simulink model "solarMomentSimplified"  (R2023b)
settings: Solver=VariableStepAuto  StartTime=0.0  StopTime=Tfinal  RelTol=1e-3
model workspace (MAT data in the model file):
  I_sim = [38538.5406483  0  0; 0  45879.2150575  0; 0  0  36244.5798954]
  areas = [26.28; 12; 3; 7.5; 17.1; 53.96; 53.96; 4.5; 26.28; 20.1]
  centroids = [4.30109589041  0  1.69726027397; 8.04  1.25  2.4; 7.44  1.25  4.8; 0  1.25  1.5; 3.42  1.25  3; 4.02  9.6  2.3; 4.02  9.6  2.3; 6.84  1.25  3.9; 4.30109589041  0  1.69726027397; 4.02  1.25  0]
  normalVectors = [0  -1  0; 1  0  0; 0  0  1; -1  0  0; 0  0  1; 0  0  1; 0  0  -1; -1  0  0; 0  1  0; 0  0  -1]
  rcm = [4.05894270882 1.95833333333 1.80412649485]
values from neighbouring files (symbols this model uses):
  A_ptob = [0.00452111179393  0.994865050863  -0.101109297888; -0.99864921572  -0.000741813086313  -0.051953764597; -0.0517619888586  0.101207609816  0.993517848971]    [magConstants.mat]
libraries: vrlib x1
settings Model: Creator=kristopherriordan  LastModifiedBy=annahylbert
settings DebuggingCC: UnderSpecifiedDimensionMsg=warning

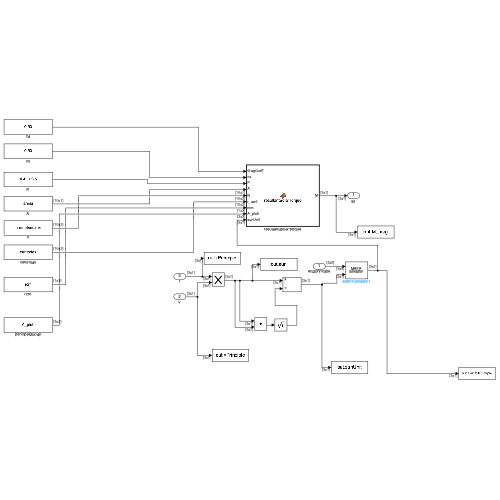
[thumbnail: Simulink's stored preview of the top-level diagram]
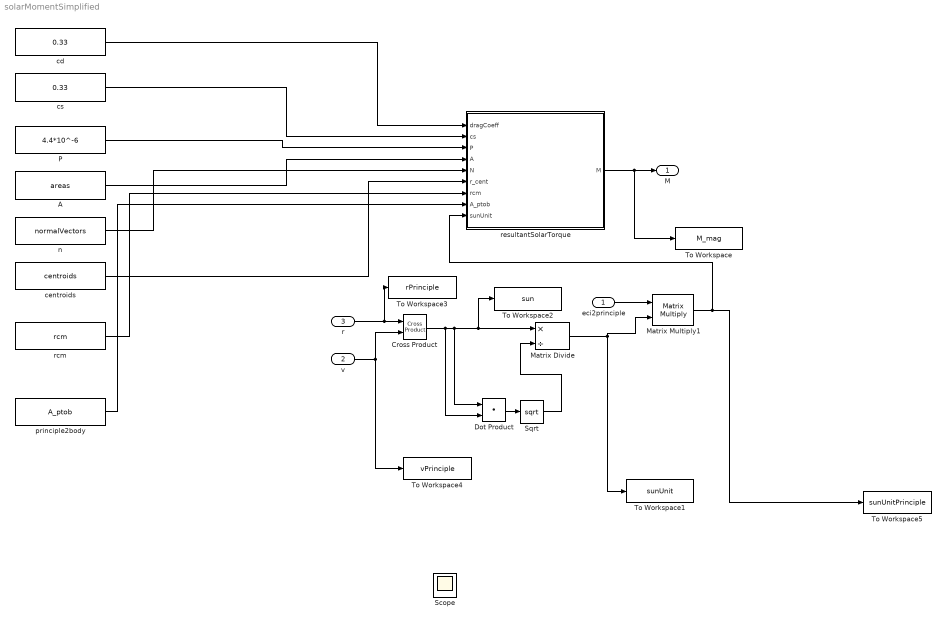
== system solarMomentSimplified ==
  eci2principle : Inport  PortDimensions=[3 3]
  v : Inport  Port=2  PortDimensions=[3 1]
  r : Inport  Port=3  PortDimensions=[3 1]
  A : Constant  Value=areas  VectorParams1D=off
  Cross Product : vrlib/Utilities/Cross Product
  Dot Product : DotProduct  OutDataTypeStr=Inherit: Inherit via internal rule
  Matrix Divide : Product  Inputs=*/
  Matrix Multiply1 : Product  Multiplication=Matrix(*)
  P : Constant  Value=4.4*10^-6  VectorParams1D=off
  Sqrt : Sqrt
  To Workspace : ToWorkspace  VariableName=M_mag  SampleTime=-1
      settings: Save2DSignal=2-D array (concatenate along first dimension)
  To Workspace1 : ToWorkspace  VariableName=sunUnit  SampleTime=-1
      settings: Save2DSignal=2-D array (concatenate along first dimension)
  To Workspace2 : ToWorkspace  VariableName=sun  SampleTime=-1
      settings: Save2DSignal=2-D array (concatenate along first dimension)
  To Workspace3 : ToWorkspace  VariableName=rPrinciple  SampleTime=-1
      settings: Save2DSignal=2-D array (concatenate along first dimension)
  To Workspace4 : ToWorkspace  VariableName=vPrinciple  SampleTime=-1
      settings: Save2DSignal=2-D array (concatenate along first dimension)
  To Workspace5 : ToWorkspace  VariableName=sunUnitPrinciple  SampleTime=-1
      settings: Save2DSignal=2-D array (concatenate along first dimension)
  cd : Constant  Value=0.33  VectorParams1D=off
  centroids : Constant  Value=centroids  VectorParams1D=off
  cs : Constant  Value=0.33  VectorParams1D=off
  n : Constant  Value=normalVectors  VectorParams1D=off
  principle2body : Constant  Value=A_ptob  VectorParams1D=off
  rcm : Constant  Value=rcm  VectorParams1D=off
  resultantSolarTorque : MATLAB Function  TreatAsAtomicUnit=on
  M : Outport
  Scope : Scope
  wires:
  centroids/1 -> resultantSolarTorque/6(r_cent)
  cd/1 -> resultantSolarTorque/1(dragCoeff)
  n/1 -> resultantSolarTorque/5(N)
  cs/1 -> resultantSolarTorque/2(cs)
  A/1 -> resultantSolarTorque/4(A)
  rcm/1 -> resultantSolarTorque/7(rcm)
  P/1 -> resultantSolarTorque/3(P)
  principle2body/1 -> resultantSolarTorque/8(A_ptob)
  Dot Product/1 -> Sqrt/1
  Sqrt/1 -> Matrix Divide/2
  resultantSolarTorque/1(M) -> To Workspace/1, M/1
  Cross Product/1 -> Dot Product/2, To Workspace2/1, Matrix Divide/1, Dot Product/1
  r/1 -> To Workspace3/1, Cross Product/1
  v/1 -> To Workspace4/1, Cross Product/2
  eci2principle/1 -> Matrix Multiply1/1
  Matrix Divide/1 -> To Workspace1/1, Matrix Multiply1/2
  Matrix Multiply1/1 -> resultantSolarTorque/9(sunUnit), To Workspace5/1

== matlab function solarMomentSimplified/resultantSolarTorque ==
  data: dragCoeff input; M output; cs input; P input; A input; N input; r_cent input; rcm input; A_ptob input; sunUnit input
function M = resultantSolarTorque(dragCoeff, cs, P, A, N, r_cent, rcm, A_ptob, sunUnit)
M = zeros([3 1]);
n = size(A, 1);

% Rotate everything to principle frame
N = transpose(N);
r_cent = transpose(r_cent);
rcm = A_ptob.' * transpose(rcm);
for i=1:n
    N(:, i) = A_ptob.' * N(:, i);
    r_cent(:, i) = A_ptob.' * r_cent(:, i);
end 

for i=1:n
    dotProduct = dot(sunUnit, N(:, i));
    if dotProduct > 0 
        if dotProduct > 1 
            dotProduct = 1.00;
        end
        theta = acos(dotProduct);
        sun_force = -P*A(i)*cos(theta)*(1-cs).*sunUnit;
        normal_force = -P*A(i)*cos(theta)*2*(cs*cos(theta) + ((1/3)*dragCoeff)).*N(:,i);
        total_force = sun_force + normal_force;
        % M = M + cross(r_cent(:, i) - rcm, total_force);
        M = M + cross(r_cent(:, 3) - rcm, total_force);
    end
end
end
